simulink model "Upgrade3"  (R2017a)
settings: Solver=FixedStepDiscrete  StartTime=0.0  StopTime=2700000  RelTol=1e-3
model workspace: external: MAT-File upgradeParams.mat (data not in the file)
values from neighbouring files (symbols this model uses):
  ambulance_speed = 60    [upgradeParams.mat]
  delayConstant = 0.25    [upgradeParams.mat]
  hospital_dist = 10    [upgradeParams.mat]
  radius = 15    [upgradeParams.mat]
  transfer_lag = 50    [upgradeParams.mat]
undefined symbols (not defined in the file or in its folder): entity, m, n, readTimer
libraries: sldelib x1
(part 1 of 3)
settings Model: PauseTimes=19000  Creator=minervazhou  LastModifiedBy=minervazhou

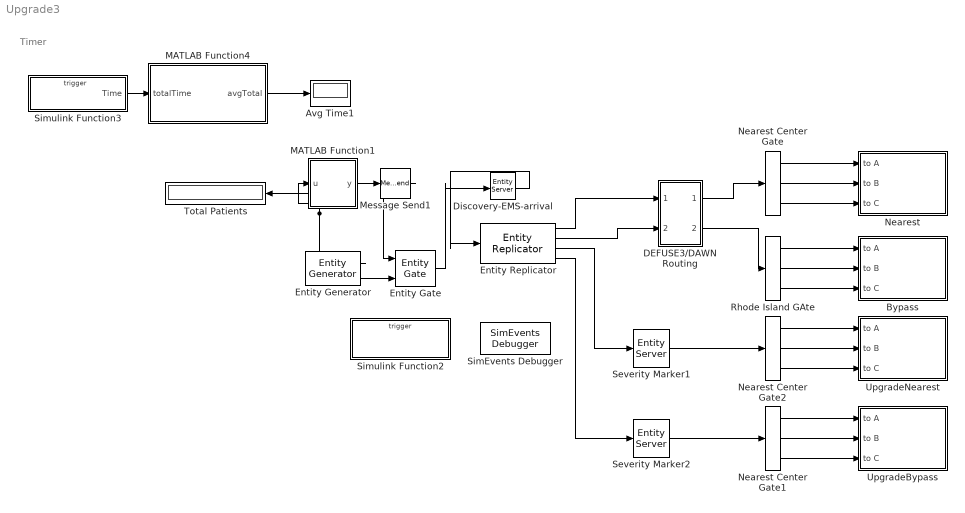
== system Upgrade3 ==
  note: Timer
  Avg Time1 : Display
  Bypass : Subsystem
  DEFUSE3/DAWN Routing : Subsystem
  Discovery-EMS-arrival : EntityServer  InputPortMessageModes=m  OutputPortMessageModes=m  Capacity=50  ServiceTimeValue=delayConstant*radius
  Entity Gate : EntityGate  InputPortMessageModes=m,m  OutputPortMessageModes=m  OpenGateAtSimulationStart=on
  Entity Generator : EntityGenerator  OutputPortMessageModes=n,m  TimeSource=MATLAB action  IntergenerationTimeAction=dt = rand(1,1)*144;  GenerateAction=|  AttributeName=NIHSS|aDistance|bDistance|tPA|tPAresponse|startTime|whichPort|CTA|LVO|onset|firstArrival|tPAtime|thromTime|ICHresp|tPAcontra|thromContra|outcomeType|throm|thromSuccess|ID|transfer|outcome|randOutcome|DAWN|unwitnessed|cDistance|firstHosp|cPop|totalTime  AttributeInitialValue=1|1|1|false|1|1|0|false|false|1|0|0|0|1|1|1|0|false|1|1|false|7|1|0|false|1|0|false|1  NumberEntitiesDeparted=on  EntityType=Structured  EntityTypeName=Entity
      | persistent next_id
      | if isempty(next_id)
      |     next_id = 1;
      |     rng(seed);
      | end
      | entity.ID = next_id;
      | next_id = next_id + 1;
      | 
      | %assign NIHSS score from set distribution
      | entity.NIHSS = randsample(0:20, 1, true, NIHSS_distribution);
      | 
      | %randomly generate a tPAresponse for later
      | entity.tPAresponse = rand();
      | %randomly generate a reperfusion success;
      | entity.thromSuccess = rand();
      | %randomly generate a ICH rate for later
      | entity.ICHresp = rand();
      | %randomly generate contraindications rate for tPA
      | entity.tPAcontra = rand();
      | %randomly generate contraindications rate for thrombectomy
      | entity.thromContra = rand();
      | entity.randOutcome = rand();
      | %DEFUSE/DAWN eligibility parameter
      | entity.DAWN = rand();
      | 
      | %given NIHSS, determine if have LVO from given prob distribution
      | LVOnum = rand();
      | if LVOnum < LVO_distribution(entity.NIHSS+1)
      |     entity.LVO=true;
      | end
      | 
      | %delay time from symptom onset to EMS arrival
      | %onset_dist = onset_flat;
      | onset_dist = onset_dist24;
      | onsetNum = rand();
      | if onsetNum <= .686
      |     %68.6% discovered automatically
      |     entity.onset = 0;
      | else
      |     %unwitnessed, assign using last known normal dist
      |     entity.unwitnessed = true;
      |     h=find(onset_dist(:)<onsetNum);
      |     if length(h)==5
      |         %12-24
      |         entity.onset=randi([720 1440]);
      |     elseif length(h)==4
      |         %6-12
      |         entity.onset=randi([360 720]);
      |     elseif length(h)==3
      |         %4.5-6 hours
      |         entity.onset=randi([270 360]);
      |     elseif length(h)==2
      |         %3-4.5 hours
      |         entity.onset=randi([180 270]);
      |     elseif length(h)==1
      |         %0-3 hours
      |         entity.onset=randi(180);
      |     end
      | end
      | 
      | %center is at (0,0)
      | %hospitals in equilateral triangle with length hospital_dist
      | hosA = [-hospital_dist/2, -hospital_dist/(2*sqrt(3))];
      | hosC = [hospital_dist/2, -hospital_dist/(2*sqrt(3))];
      | hosB = [0, hospital_dist/sqrt(3)];
      | %determine where pt appears
      | pt_x = ((2*radius)*rand())-radius;
      | pt_y = ((2*radius)*rand())-radius;
      | while sqrt(pt_x^2+pt_y^2)>radius
      |     pt_x = ((2*radius)*rand())-radius;
      |     pt_y = ((2*radius)*rand())-radius;
      | end
      | 
      | %ambulance moving at set speed = 60 mph
      | %in minutes
      | entity.aDistance = sqrt((hosA(1)-pt_x)^2 + (hosA(2)-pt_y)^2)*(60/ambulance_speed);
      | entity.bDistance = sqrt((hosB(1)-pt_x)^2 + (hosB(2)-pt_y)^2)*(60/ambulance_speed);
      | entity.cDistance = sqrt((hosC(1)-pt_x)^2 + (hosC(2)-pt_y)^2)*(60/ambulance_speed);
      | 
      | lengths = [entity.aDistance, entity.bDistance, entity.cDistance];
      | minL = find(lengths==min(lengths));
      | entity.whichPort = minL(randi(length(minL)));
      | 
      | if entity.whichPort ==3
      |     entity.cPop = true;
      | end
      settings: OutputPortMap=o0,o3
  Entity Replicator : EntityReplicator  InputPortMessageModes=m  OutputPortMessageModes=m,m,m,m  NumberReplicas=3
      settings: OutputPortMap=o0,o1,o2,o3
  MATLAB Function1 : MATLAB Function  TreatAsAtomicUnit=on
  MATLAB Function4 : MATLAB Function  TreatAsAtomicUnit=on
  Message Send1 : MessageSend  OutputPortMessageModes=m
      settings: InputPortMap=u1
  Nearest : Subsystem
  Nearest Center Gate : EntityOutputSwitch  InputPortMessageModes=m  OutputPortMessageModes=m,m,m  NumberOutputPorts=3  SwitchingCriterion=From attribute  SwitchAttributeName=whichPort
      settings: OutputPortMap=o0,o1,o2
  Nearest Center Gate1 : EntityOutputSwitch  InputPortMessageModes=m  OutputPortMessageModes=m,m,m  NumberOutputPorts=3  SwitchingCriterion=From attribute  SwitchAttributeName=whichPort
      settings: OutputPortMap=o0,o1,o2
  Nearest Center Gate2 : EntityOutputSwitch  InputPortMessageModes=m  OutputPortMessageModes=m,m,m  NumberOutputPorts=3  SwitchingCriterion=From attribute  SwitchAttributeName=whichPort
      settings: OutputPortMap=o0,o1,o2
  Rhode Island GAte : EntityOutputSwitch  InputPortMessageModes=m  OutputPortMessageModes=m,m,m  NumberOutputPorts=3  SwitchingCriterion=From attribute  SwitchAttributeName=whichPort
      settings: OutputPortMap=o0,o1,o2
  Severity Marker1 : EntityServer  InputPortMessageModes=m  OutputPortMessageModes=m  Capacity=1  ServiceTimeSource=Attribute  ServiceTimeValue=0  ServiceTimeAttributeName=onset  EntryAction=entity.startTime = startTimer();
  Severity Marker2 : EntityServer  InputPortMessageModes=m  OutputPortMessageModes=m  Capacity=1  ServiceTimeSource=Attribute  ServiceTimeValue=0  ServiceTimeAttributeName=onset  EntryAction=|
      | if entity.NIHSS >= severe_cutoff
      |     if entity.whichPort==2
      |         if entity.aDistance<=entity.cDistance
      |             entity.whichPort=1;
      |         else
      |             entity.whichPort=3;
      |         end
      |     end
      | end
      | entity.startTime = startTimer();
  SimEvents Debugger : sldelib/SimEvents Debugger  EnableDebugger=on  ShowInLibBrowser=0
      settings: SourceProductName=SimEvents  SourceProductBaseCode=SE
  Simulink Function2 : Subsystem  TreatAsAtomicUnit=on
  Simulink Function3 : Subsystem  TreatAsAtomicUnit=on
  Total Patients : Display
  UpgradeBypass : Subsystem
  UpgradeNearest : Subsystem
  wires:
  Entity Generator/1 -> MATLAB Function1/1(u), Total Patients/1
  Nearest Center Gate/1 -> Nearest/1(to A)
  Nearest Center Gate/2 -> Nearest/2(to B)
  Rhode Island GAte/1 -> Bypass/1(to A)
  Rhode Island GAte/2 -> Bypass/2(to B)
  DEFUSE3/DAWN Routing/1(Out2) -> Nearest Center Gate/1
  DEFUSE3/DAWN Routing/2(Out4) -> Rhode Island GAte/1
  MATLAB Function1/1(y) -> Message Send1/1
  Entity Generator/2 -> Entity Gate/2
  Message Send1/1 -> Entity Gate/1
  Simulink Function3/1(Time) -> MATLAB Function4/1(totalTime)
  MATLAB Function4/1(avgTotal) -> Avg Time1/1
  Entity Gate/1 -> Discovery-EMS-arrival/1
  Discovery-EMS-arrival/1 -> Entity Replicator/1
  Nearest Center Gate/3 -> Nearest/3(to C)
  Rhode Island GAte/3 -> Bypass/3(to C)
  Nearest Center Gate2/2 -> UpgradeNearest/2(to B)
  Nearest Center Gate2/1 -> UpgradeNearest/1(to A)
  Severity Marker1/1 -> Nearest Center Gate2/1
  Nearest Center Gate2/3 -> UpgradeNearest/3(to C)
  Nearest Center Gate1/3 -> UpgradeBypass/3(to C)
  Severity Marker2/1 -> Nearest Center Gate1/1
  Nearest Center Gate1/1 -> UpgradeBypass/1(to A)
  Nearest Center Gate1/2 -> UpgradeBypass/2(to B)
  Entity Replicator/1 -> DEFUSE3/DAWN Routing/1(In2)
  Entity Replicator/2 -> DEFUSE3/DAWN Routing/2(In4)
  Entity Replicator/3 -> Severity Marker1/1
  Entity Replicator/4 -> Severity Marker2/1

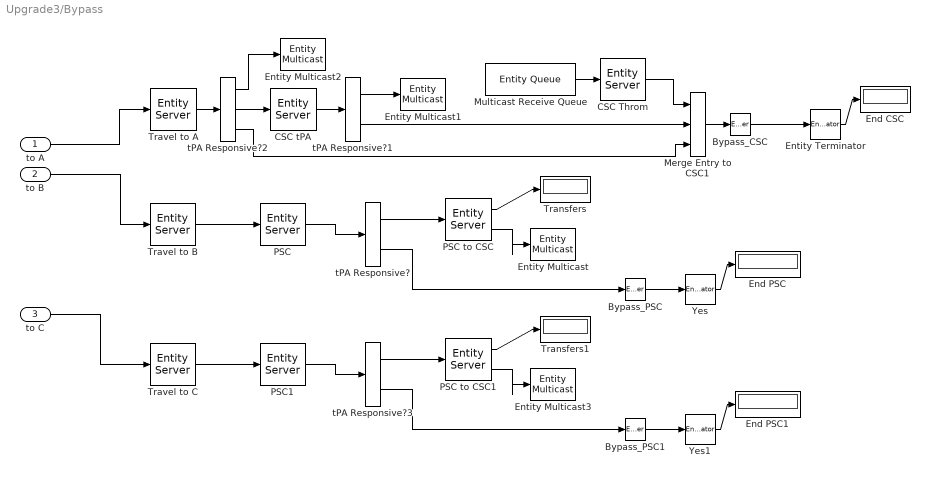
== system Upgrade3/Bypass ==
  to A : Inport
  to B : Inport  Port=2
  to C : Inport  Port=3
  Bypass_CSC : EntityServer  InputPortMessageModes=m  OutputPortMessageModes=m  Capacity=inf  ServiceTimeValue=0  EntryAction=|
      | entity.totalTime = startTimer() - entity.startTime;
      | 
      | if entity.LVO
      |     if entity.outcomeType == 1
      |         if entity.totalTime <=360
      |             dist = NT_LVO;
      |         elseif entity.unwitnessed
      |             if entity.totalTime <=960
      |                 dist = MT_DEFUSE3unknown;
      |             else
      |                 dist = MT_DAWNunknown;
      |             end
      |         elseif entity.totalTime <=960
      |             %witnessed and 6-16 hrs
      |             dist = MT_DEFUSE3witnessed;
      |         else
      |             %witnessed and 16-24 hrs
      |             dist = MT_DAWNwitnessed;
      |         end
      |     elseif entity.outcomeType == 2
      |         if entity.tPAtime <=360
      |             dist = tPA_LVO;
      |         else
      |             dist = NT_LVO;
      |         end
      |     elseif entity.outcomeType == 3 | entity.outcomeType ==4
      |         if entity.thromTime <= 180
      |             dist = throm_180;
      |         elseif entity.thromTime <=240
      |             dist = throm_240;
      |         elseif entity.thromTime <=300
      |             dist = throm_300;
      |         elseif entity.thromTime <=360
      |             dist = throm_360;
      |         elseif entity.unwitnessed
      |             if entity.thromTime <=960
      |                 dist = EVT_DEFUSE3unknown;
      |             else
      |                 dist = EVT_DAWNunknown;
      |             end
      |         elseif entity.thromTime <=960
      |             %witnessed and 6-16 hrs
      |             dist = EVT_DEFUSE3witnessed;
      |         else
      |             %witnessed and 16-24 hrs
      |             dist = EVT_DAWNwitnessed;
      |         end
      |     else
      |         dist = [];
      |     end
      | else
      |     if entity.outcomeType==1
      |         if entity.firstArrival <= 90
      |             dist = NT_90;
      |         elseif entity.firstArrival <= 180
      |             dist = NT_180;
      |         elseif entity.firstArrival <= 270
      |             dist = NT_270;
      |         else
      |             dist = NT_360;
      |         end
      |     elseif entity.outcomeType==2
      |         if entity.firstArrival <= 90
      |             dist = tPA_90;
      |         elseif entity.firstArrival <= 180
      |             dist = tPA_180;
      |         elseif entity.firstArrival <= 270
      |             dist = tPA_270;
      |         else
      |             dist = tPA_360;
      |         end
      |     else
      |         dist = [];
      |     end
      | end
      | if isempty(dist)
      |     entity.outcome = 999; %error message basically
      | else
      |     b = find(dist(:)<entity.randOutcome);
      |     if isempty(b)
      |         entity.outcome=0;
      |     else
      |         entity.outcome = b(length(b));
      |     end
      | end
  Bypass_PSC : EntityServer  InputPortMessageModes=m  OutputPortMessageModes=m  Capacity=inf  ServiceTimeValue=0  EntryAction=|
      | entity.totalTime = startTimer() - entity.startTime;
      | 
      | if entity.LVO
      |     if entity.outcomeType == 1
      |         if entity.totalTime <=360
      |             dist = NT_LVO;
      |         elseif entity.unwitnessed
      |             if entity.totalTime <=960
      |                 dist = MT_DEFUSE3unknown;
      |             else
      |                 dist = MT_DAWNunknown;
      |             end
      |         elseif entity.totalTime <=960
      |             %witnessed and 6-16 hrs
      |             dist = MT_DEFUSE3witnessed;
      |         else
      |             %witnessed and 16-24 hrs
      |             dist = MT_DAWNwitnessed;
      |         end
      |     elseif entity.outcomeType == 2
      |         if entity.tPAtime <=360
      |             dist = tPA_LVO;
      |         else
      |             dist = NT_LVO;
      |         end
      |     elseif entity.outcomeType == 3 | entity.outcomeType ==4
      |         if entity.thromTime <= 180
      |             dist = throm_180;
      |         elseif entity.thromTime <=240
      |             dist = throm_240;
      |         elseif entity.thromTime <=300
      |             dist = throm_300;
      |         elseif entity.thromTime <=360
      |             dist = throm_360;
      |         elseif entity.unwitnessed
      |             if entity.thromTime <=960
      |                 dist = EVT_DEFUSE3unknown;
      |             else
      |                 dist = EVT_DAWNunknown;
      |             end
      |         elseif entity.thromTime <=960
      |             %witnessed and 6-16 hrs
      |             dist = EVT_DEFUSE3witnessed;
      |         else
      |             %witnessed and 16-24 hrs
      |             dist = EVT_DAWNwitnessed;
      |         end
      |     else
      |         dist = [];
      |     end
      | else
      |     if entity.outcomeType==1
      |         if entity.firstArrival <= 90
      |             dist = NT_90;
      |         elseif entity.firstArrival <= 180
      |             dist = NT_180;
      |         elseif entity.firstArrival <= 270
      |             dist = NT_270;
      |         else
      |             dist = NT_360;
      |         end
      |     elseif entity.outcomeType==2
      |         if entity.firstArrival <= 90
      |             dist = tPA_90;
      |         elseif entity.firstArrival <= 180
      |             dist = tPA_180;
      |         elseif entity.firstArrival <= 270
      |             dist = tPA_270;
      |         else
      |             dist = tPA_360;
      |         end
      |     else
      |         dist = [];
      |     end
      | end
      | if isempty(dist)
      |     entity.outcome = 999; %error message basically
      | else
      |     b = find(dist(:)<entity.randOutcome);
      |     if isempty(b)
      |         entity.outcome=0;
      |     else
      |         entity.outcome = b(length(b));
      |     end
      | end
  Bypass_PSC1 : EntityServer  InputPortMessageModes=m  OutputPortMessageModes=m  Capacity=inf  ServiceTimeValue=0  EntryAction=|
      | entity.totalTime = startTimer() - entity.startTime;
      | 
      | if entity.LVO
      |     if entity.outcomeType == 1
      |         if entity.totalTime <=360
      |             dist = NT_LVO;
      |         elseif entity.unwitnessed
      |             if entity.totalTime <=960
      |                 dist = MT_DEFUSE3unknown;
      |             else
      |                 dist = MT_DAWNunknown;
      |             end
      |         elseif entity.totalTime <=960
      |             %witnessed and 6-16 hrs
      |             dist = MT_DEFUSE3witnessed;
      |         else
      |             %witnessed and 16-24 hrs
      |             dist = MT_DAWNwitnessed;
      |         end
      |     elseif entity.outcomeType == 2
      |         if entity.tPAtime <=360
      |             dist = tPA_LVO;
      |         else
      |             dist = NT_LVO;
      |         end
      |     elseif entity.outcomeType == 3 | entity.outcomeType ==4
      |         if entity.thromTime <= 180
      |             dist = throm_180;
      |         elseif entity.thromTime <=240
      |             dist = throm_240;
      |         elseif entity.thromTime <=300
      |             dist = throm_300;
      |         elseif entity.thromTime <=360
      |             dist = throm_360;
      |         elseif entity.unwitnessed
      |             if entity.thromTime <=960
      |                 dist = EVT_DEFUSE3unknown;
      |             else
      |                 dist = EVT_DAWNunknown;
      |             end
      |         elseif entity.thromTime <=960
      |             %witnessed and 6-16 hrs
      |             dist = EVT_DEFUSE3witnessed;
      |         else
      |             %witnessed and 16-24 hrs
      |             dist = EVT_DAWNwitnessed;
      |         end
      |     else
      |         dist = [];
      |     end
      | else
      |     if entity.outcomeType==1
      |         if entity.firstArrival <= 90
      |             dist = NT_90;
      |         elseif entity.firstArrival <= 180
      |             dist = NT_180;
      |         elseif entity.firstArrival <= 270
      |             dist = NT_270;
      |         else
      |             dist = NT_360;
      |         end
      |     elseif entity.outcomeType==2
      |         if entity.firstArrival <= 90
      |             dist = tPA_90;
      |         elseif entity.firstArrival <= 180
      |             dist = tPA_180;
      |         elseif entity.firstArrival <= 270
      |             dist = tPA_270;
      |         else
      |             dist = tPA_360;
      |         end
      |     else
      |         dist = [];
      |     end
      | end
      | if isempty(dist)
      |     entity.outcome = 999; %error message basically
      | else
      |     b = find(dist(:)<entity.randOutcome);
      |     if isempty(b)
      |         entity.outcome=0;
      |     else
      |         entity.outcome = b(length(b));
      |     end
      | end
  CSC Throm : EntityServer  InputPortMessageModes=m  OutputPortMessageModes=m  Capacity=2  ServiceTimeSource=MATLAB action  ServiceTimeValue=CSC_NTP  ServiceTimeAction=|  ServiceCompleteAction=|
      ServiceTimeAction=|
      | if ~entity.CTA
      |     %did respond to tPA or have hemorrhage
      |     %then only did CTA and discovered no go
      |     if entity.tPA && ((entity.tPAresponse < tPAresp_LVO) | (entity.ICHresp < ICHrate))
      |         dt = CTA_time;
      |     else
      |         dt = CTA_time + CSC_NTP;
      |     end
      | else
      |     dt = CSC_NTP;
      | end
      ServiceCompleteAction=|
      | if ~entity.CTA
      |     entity.CTA=true;
      | end
      | 
      | if entity.throm
      |     %if previously already decided should have thrombectomy
      |     %outcomeType already assigned
      |     entity.thromTime = startTimer() - entity.startTime;
      | elseif ~entity.tPA
      |     %bypassed tPA in CSC
      |     entity.throm = true;
      |     entity.thromTime = startTimer() - entity.startTime;
      |     entity.outcomeType = 3;
      | elseif (entity.tPAresponse >= tPAresp_LVO) && (entity.ICHresp > ICHrate)
      |     %did not respond tPA and did not hemorrhage
      |     entity.throm = true;
      |     entity.thromTime = startTimer() - entity.startTime;
      |     entity.outcomeType = 4;
      | else
      |     %responded to tPA
      |     entity.outcomeType = 2;
      | end
      | 
      | %if had thrombectomy and did not successfully recanalize
      | if entity.throm && entity.thromSuccess > reperf_rate
      |     if entity.outcomeType == 3
      |         entity.outcomeType = 1;
      |     elseif entity.outcomeType == 4
      |         entity.outcomeType = 2;
      |     end
      | end
  CSC tPA : EntityServer  InputPortMessageModes=m  OutputPortMessageModes=m  Capacity=75  ServiceTimeValue=CSC_DTN  ServiceCompleteAction=|
      | entity.tPA = true;
      | entity.tPAtime = startTimer() - entity.startTime;
      | current = entity.tPAtime;
      | 
      | %if has LVO, no throm contraindications, and above min cutoff
      | if entity.LVO && (entity.thromContra > throm_CI) && entity.NIHSS >= throm_min
      |     %don't care if respond to tPA, immediately to thrombectomy
      |     entity.whichPort = 1;
      | else
      |     entity.whichPort = 2;
      |     entity.outcomeType = 2;
      | end
  End CSC : Display
  End PSC : Display
  End PSC1 : Display
  Entity Multicast{,1..3} (4 alike) : EntityMulticast  InputPortMessageModes=m  MulticastTag=Bypass_throm
  Entity Terminator : EntityTerminator  InputPortMessageModes=m  EntryAction=readTimer(entity.totalTime);  NumberEntitiesArrived=on
      settings: OutputPortMap=o0
  Merge Entry to CSC1 : EntityInputSwitch  InputPortMessageModes=m,m,m  OutputPortMessageModes=m  NumberInputPorts=3
      settings: InputPortMap=u1,u2,u3
  Multicast Receive Queue : EntityQueue  OutputPortMessageModes=m  Capacity=100  EntityArrivalSource=Multicast  MulticastTag=Bypass_throm
      settings: OutputPortMap=o5
  PSC : EntityServer  InputPortMessageModes=m  OutputPortMessageModes=m  Capacity=50  ServiceTimeSource=MATLAB action  ServiceTimeValue=PSC_DTN  ServiceTimeAction=|  ServiceCompleteAction=|
      ServiceTimeAction=|
      | %no contraindications for tPA
      | if entity.tPAcontra > tPA_CI && (entity.firstArrival <= tPA_cutoff)
      |     if entity.LVO && PSC_CTA && (entity.tPAresponse > tPAresp_LVO) && (entity.ICHresp > ICHrate)
      |         dt = PSC_DTN + CTA_time;
      |     else
      |         dt = PSC_DTN;
      |     end
      | else
      |     if entity.LVO && PSC_CTA
      |         dt = CTA_time;
      |     else
      |         dt = 0;
      |     end
      | end
      ServiceCompleteAction=|
      | current = startTimer() - entity.startTime;
      | 
      | %get tPA if no contraindications and less than 4.5 hours
      | if (entity.tPAcontra > tPA_CI) && (entity.firstArrival <= tPA_cutoff)
      |     entity.tPA = true;
      |     entity.tPAtime = startTimer() - entity.startTime;
      |     if entity.LVO && (entity.thromContra > throm_CI) && (entity.tPAresponse > tPAresp_LVO) && (entity.ICHresp > ICHrate) && entity.NIHSS >= throm_min
      |         %has LVO, didn't respond to tPA, no contraindications, no hemorrhage, above min NIHSS
      |         entity.whichPort = 1;
      |         entity.outcomeType = 4;
      |         entity.throm = true;
      |     else
      |         %no LVO, responded to tPA, hemorrhaged or has throm contraindications
      |         entity.whichPort = 2;
      |         entity.outcomeType = 2;
      |     end
      | else    
      | %no tPA
      |     if entity.LVO && (entity.NIHSS >= throm_min) && (((current + hospital_dist <= HERMES_cutoff) && (entity.thromContra > throm_CI)) | ((current + hospital_dist <= DEFUSE_cutoff) && (entity.DAWN <= DEFUSEe)) | ((current + hospital_dist <= DAWN_cutoff) && (entity.DAWN <= DAWNe) && (entity.NIHSS >= DAWN_NIHSS_min)))
      |         %ineligible for tPA but still eligible for thrombectomy
      |         entity.whichPort = 1;
      |         entity.outcomeType = 3;
      |         entity.throm = true;    
      |     else
      |     %no treatment
      |         entity.whichPort = 2;
      |         entity.outcomeType = 1;
      |     end
      | end
      | 
      | if PSC_CTA
      |     entity.CTA=true;
      | end
  PSC to CSC : EntityServer  InputPortMessageModes=m  OutputPortMessageModes=n,m  Capacity=75  ServiceTimeValue=((hospital_dist/ambulance_speed)*60)+transfer_lag  ServiceCompleteAction=|  NumberEntitiesDeparted=on
      | entity.throm = true;
      | entity.transfer = true;
      settings: OutputPortMap=o0,o9
  PSC to CSC1 : EntityServer  InputPortMessageModes=m  OutputPortMessageModes=n,m  Capacity=75  ServiceTimeValue=((hospital_dist/ambulance_speed)*60)+transfer_lag  ServiceCompleteAction=|  NumberEntitiesDeparted=on
      | entity.throm = true;
      | entity.transfer = true;
      settings: OutputPortMap=o0,o9
  PSC1 : EntityServer  InputPortMessageModes=m  OutputPortMessageModes=m  Capacity=50  ServiceTimeSource=MATLAB action  ServiceTimeValue=PSC_DTN  ServiceTimeAction=|  ServiceCompleteAction=|
      ServiceTimeAction=|
      | %no contraindications for tPA
      | if entity.tPAcontra > tPA_CI && (entity.firstArrival <= tPA_cutoff)
      |     if entity.LVO && PSC_CTA && (entity.tPAresponse > tPAresp_LVO) && (entity.ICHresp > ICHrate)
      |         dt = PSC_DTN + CTA_time;
      |     else
      |         dt = PSC_DTN;
      |     end
      | else
      |     if entity.LVO && PSC_CTA
      |         dt = CTA_time;
      |     else
      |         dt = 0;
      |     end
      | end
      ServiceCompleteAction=|
      | current = startTimer() - entity.startTime;
      | 
      | %get tPA if no contraindications and less than 4.5 hours
      | if (entity.tPAcontra > tPA_CI) && (entity.firstArrival <= tPA_cutoff)
      |     entity.tPA = true;
      |     entity.tPAtime = startTimer() - entity.startTime;
      |     if entity.LVO && (entity.thromContra > throm_CI) && (entity.tPAresponse > tPAresp_LVO) && (entity.ICHresp > ICHrate) && entity.NIHSS >= throm_min
      |         %has LVO, didn't respond to tPA, no contraindications, no hemorrhage, above min NIHSS
      |         entity.whichPort = 1;
      |         entity.outcomeType = 4;
      |         entity.throm = true;
      |     else
      |         %no LVO, responded to tPA, hemorrhaged or has throm contraindications
      |         entity.whichPort = 2;
      |         entity.outcomeType = 2;
      |     end
      | else    
      | %no tPA
      |     if entity.LVO && (entity.NIHSS >= throm_min) && (((current + hospital_dist <= HERMES_cutoff) && (entity.thromContra > throm_CI)) | ((current + hospital_dist <= DEFUSE_cutoff) && (entity.DAWN <= DEFUSEe)) | ((current + hospital_dist <= DAWN_cutoff) && (entity.DAWN <= DAWNe) && (entity.NIHSS >= DAWN_NIHSS_min)))
      |         %ineligible for tPA but still eligible for thrombectomy
      |         entity.whichPort = 1;
      |         entity.outcomeType = 3;
      |         entity.throm = true;    
      |     else
      |     %no treatment
      |         entity.whichPort = 2;
      |         entity.outcomeType = 1;
      |     end
      | end
      | 
      | if PSC_CTA
      |     entity.CTA=true;
      | end
  Transfers : Display
  Transfers1 : Display
  Travel to A : EntityServer  InputPortMessageModes=m  OutputPortMessageModes=m  Capacity=75  ServiceTimeSource=Attribute  ServiceTimeValue=cscDis  ServiceTimeAttributeName=aDistance  EntryAction=entity.firstHosp = 1;  ServiceCompleteAction=|
      | %time exceeds 4.5 hours then bypass tPA
      | %exceeds 24 hours then no thrombectomy
      | current = startTimer()-entity.startTime;
      | 
      | %past 24 hours
      | if current >= DAWN_cutoff
      |     entity.whichPort = 3;
      |     entity.outcomeType = 1;
      | %past 4.5 hrs or have contraindications, no tPA
      | elseif (current >= tPA_cutoff) | (entity.tPAcontra < tPA_CI)
      |     if entity.LVO && entity.NIHSS >= throm_min && (((current <= HERMES_cutoff) && (entity.thromContra > throm_CI)) | ((current <= DEFUSE_cutoff) && (entity.DAWN <= DEFUSEe)) | ((current <= DAWN_cutoff) && (entity.DAWN <= DAWNe) && (entity.NIHSS >= DAWN_NIHSS_min)))
      |         %with LVO, no CI for thrombectomy, above min NIHSS cutoff
      |         entity.whichPort = 1;
      |         entity.throm = true;
      |         entity.outcomeType = 3;
      |     else
      |         %not eligible for tPA or thrombectomy
      |         entity.whichPort = 3;
      |         entity.outcomeType = 1;
      |     end
      | else
      |     entity.whichPort = 2;
      | end
      | 
      | entity.firstArrival = startTimer() - entity.startTime;
  Travel to B : EntityServer  InputPortMessageModes=m  OutputPortMessageModes=m  Capacity=75  ServiceTimeSource=Attribute  ServiceTimeValue=9  ServiceTimeAttributeName=bDistance  EntryAction=entity.firstHosp = 2;  ServiceCompleteAction=entity.firstArrival = startTimer() - entity.startTime;
  Travel to C : EntityServer  InputPortMessageModes=m  OutputPortMessageModes=m  Capacity=75  ServiceTimeSource=Attribute  ServiceTimeValue=9  ServiceTimeAttributeName=cDistance  EntryAction=entity.firstHosp = 3;  ServiceCompleteAction=entity.firstArrival = startTimer() - entity.startTime;
  Yes : EntityTerminator  InputPortMessageModes=m  EntryAction=readTimer(entity.totalTime);  NumberEntitiesArrived=on
      settings: OutputPortMap=o0
  Yes1 : EntityTerminator  InputPortMessageModes=m  EntryAction=readTimer(entity.totalTime);  NumberEntitiesArrived=on
      settings: OutputPortMap=o0
  tPA Responsive? : EntityOutputSwitch  InputPortMessageModes=m  OutputPortMessageModes=m,m  SwitchingCriterion=From attribute  SwitchAttributeName=whichPort
  tPA Responsive?1 : EntityOutputSwitch  InputPortMessageModes=m  OutputPortMessageModes=m,m  SwitchingCriterion=From attribute  SwitchAttributeName=whichPort
  tPA Responsive?2 : EntityOutputSwitch  InputPortMessageModes=m  OutputPortMessageModes=m,m,m  NumberOutputPorts=3  SwitchingCriterion=From attribute  SwitchAttributeName=whichPort
      settings: OutputPortMap=o0,o1,o2
  tPA Responsive?3 : EntityOutputSwitch  InputPortMessageModes=m  OutputPortMessageModes=m,m  SwitchingCriterion=From attribute  SwitchAttributeName=whichPort
  wires:
  to B/1 -> Travel to B/1
  to A/1 -> Travel to A/1
  tPA Responsive?/1 -> PSC to CSC/1
  PSC/1 -> tPA Responsive?/1
  PSC to CSC/1 -> Transfers/1
  Yes/1 -> End PSC/1
  Entity Terminator/1 -> End CSC/1
  CSC tPA/1 -> tPA Responsive?1/1
  CSC Throm/1 -> Merge Entry to CSC1/1
  PSC to CSC/2 -> Entity Multicast/1
  tPA Responsive?1/1 -> Entity Multicast1/1
  Multicast Receive Queue/1 -> CSC Throm/1
  tPA Responsive?1/2 -> Merge Entry to CSC1/2
  Travel to A/1 -> tPA Responsive?2/1
  tPA Responsive?2/1 -> Entity Multicast2/1
  tPA Responsive?2/2 -> CSC tPA/1
  tPA Responsive?2/3 -> Merge Entry to CSC1/3
  Merge Entry to CSC1/1 -> Bypass_CSC/1
  Bypass_CSC/1 -> Entity Terminator/1
  Travel to B/1 -> PSC/1
  Bypass_PSC/1 -> Yes/1
  tPA Responsive?/2 -> Bypass_PSC/1
  Travel to C/1 -> PSC1/1
  PSC to CSC1/2 -> Entity Multicast3/1
  tPA Responsive?3/2 -> Bypass_PSC1/1
  Yes1/1 -> End PSC1/1
  tPA Responsive?3/1 -> PSC to CSC1/1
  Bypass_PSC1/1 -> Yes1/1
  PSC to CSC1/1 -> Transfers1/1
  PSC1/1 -> tPA Responsive?3/1
  to C/1 -> Travel to C/1

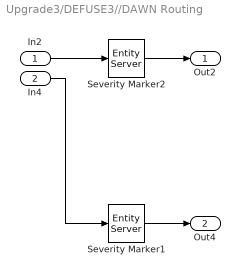
== system Upgrade3/DEFUSE3//DAWN Routing ==
  In2 : Inport
  In4 : Inport  Port=2
  Severity Marker1 : EntityServer  InputPortMessageModes=m  OutputPortMessageModes=m  Capacity=1  ServiceTimeSource=Attribute  ServiceTimeValue=0  ServiceTimeAttributeName=onset  EntryAction=|
      | if entity.NIHSS >= severe_cutoff
      |     entity.whichPort = 1;
      | end
      | entity.startTime = startTimer();
  Severity Marker2 : EntityServer  InputPortMessageModes=m  OutputPortMessageModes=m  Capacity=1  ServiceTimeSource=Attribute  ServiceTimeValue=0  ServiceTimeAttributeName=onset  EntryAction=entity.startTime = startTimer();
  Out2 : Outport
  Out4 : Outport  Port=2
  wires:
  Severity Marker2/1 -> Out2/1
  In2/1 -> Severity Marker2/1
  Severity Marker1/1 -> Out4/1
  In4/1 -> Severity Marker1/1
